simulink model "SR26_2024a"  (R2024a)
settings: Solver=FixedStepDiscrete  StartTime=0.0  StopTime=10.0  FixedStep=0.01  RelTol=1e-3  EnableMultiTasking=on
PreLoadFcn:
  | try, model_open; catch, disp('Error occurred while executing model pre-load callback: model_open.m'); disp('Please assure that the MATLAB working directory is set to the model directory before opening.'); end
InitFcn:
  | try, model_open; catch, end
values from neighbouring files (symbols this model uses):
  dt = 10.0    [SR26.sldd]
undefined symbols (not defined in the file or in its folder): GCM, raptor_get_safe_string, raptor_xcp_function
libraries: Raptor_lib x42, Utilities x6, simulink x5, IO x5, APPS_BSPC x4, Cooling x3, StateMachine x2, TorqueCommand x2, ATCC x2, BrakePressure x2, ThrottlePosition x2, Brakes x1
(part 1 of 2)
CloseFcn:
  | try, model_close; catch, end
settings Model: DataDictionary=SR26.sldd  Raptor_Target=GCM-1793-196-1503  Raptor_Calloc=NonVolatile (EEPROM)  RaptorUIDSize=4  RaptorBuildNum=0  Raptor_ecuaddr=11  RaptorFaultManager=Standard  RaptorFaultManagerAddXYCounts=1  Creator=hyuga  LastModifiedBy=hyuga
settings SolverCC: AlgebraicLoopSolver=TrustRegion
settings DataIOCC: LimitDataPoints=on  SaveFormat=Array  SignalLoggingSaveFormat=ModelDataLogs  ReturnWorkspaceOutputs=off
settings OptimizationCC: DefaultParameterBehavior=Inlined  ExpressionDepthLimit=2147483647  InitFltsAndDblsToZero=on  LifeSpan=1  EfficientTunableParamExpr=on
settings DebuggingCC: SolverPrmCheckMsg=warning  InheritedTsInSrcMsg=none  FcnCallInpInsideContextMsg=warning  UnconnectedInputMsg=warning  UnconnectedOutputMsg=warning  UnconnectedLineMsg=warning  StateNameClashWarn=warning  SFUnexpectedBacktrackingDiag=warning  SFNoUnconditionalDefaultTransitionDiag=warning  SFExecutionAtInitializationDiag=none  ArithmeticOperatorsInVariantConditions=warning
settings HardwareCC: ProdBitPerPointer=32  ProdBitPerSizeT=32  ProdBitPerPtrDiffT=32  ProdLargestAtomicFloat=None  ProdWordSize=32  ProdHWDeviceType=Infineon->TriCore  TargetBitPerPointer=64  TargetBitPerSizeT=64  TargetBitPerPtrDiffT=64  TargetLongLongMode=on  TargetIntDivRoundTo=Zero  TargetEndianess=LittleEndian  TargetWordSize=64  TargetHWDeviceType=MATLAB Host  ProdEqTarget=off
settings ModelReferenceCC: EnableRefExpFcnMdlSchedulingChecks=on  PropagateSignalLabelsOutOfModel=off
settings SFSimCC: SimUseLocalCustomCode=off  MATLABDynamicMemAlloc=off  CustomCodeUndefinedFunction=UseInterfaceOnly
settings RTWCC: Description=Raptor (tm)  SystemTargetFile=raptor.tlc  MakeCommand=raptor_make_rtw  TemplateMakefile=raptor.tmf  RTWUseLocalCustomCode=off  GPUComputeCapability=3.5  DLArmComputeVersion=19.05
settings CodeAppCC: IgnoreCustomStorageClasses=off  MaxIdLength=100  CustomSymbolStrType=$N$R$M  StateflowObjectComments=on  InternalIdentifier=Classic
settings STFCustomTargetCC: TargetLangStandard=C89/C90 (ANSI)  CodeReplacementLibrary=GCM196-specific  GenerateSampleERTMain=on  ModelReferenceCompliant=off  CombineOutputUpdateFcns=on  ERTCustomFileBanners=on  SupportContinuousTime=off  SupportNonInlinedSFcns=off  RemoveResetFunc=on  MATLABClassNameForMDSCustomization=Simulink.SoftwareTarget.ERTCustomization  GRTInterface=off  UseToolchainInfoCompliant=off  SystemTargetFile=raptor.tlc
settings ERTTargetCC: CodeReplacementLibrary=GCM196-specific  MultiwordLength=2048  GenerateSampleERTMain=on  ModelReferenceCompliant=off  ParMdlRefBuildCompliant=off  CompOptLevelCompliant=off  ConcurrentExecutionCompliant=off  ModelStepFunctionPrototypeControlCompliant=off  CPPClassGenCompliant=off  UseToolchainInfoCompliant=off  ExtModeMexFile=noextcomm  InlinedParameterPlacement=NonHierarchical  ERTCustomFileTemplate=example_file_process.tlc  ConvertIfToSwitch=off  SuppressUnreachableDefaultCases=off
settings ConfigComp: CovMetricSettings=dw  CovSaveCumulativeToWorkspaceVar=on  CovSaveSingleToWorkspaceVar=on  CovExternalEMLEnable=off  CovSFcnEnable=off  CovBoundaryAbsTol=1.0e-5

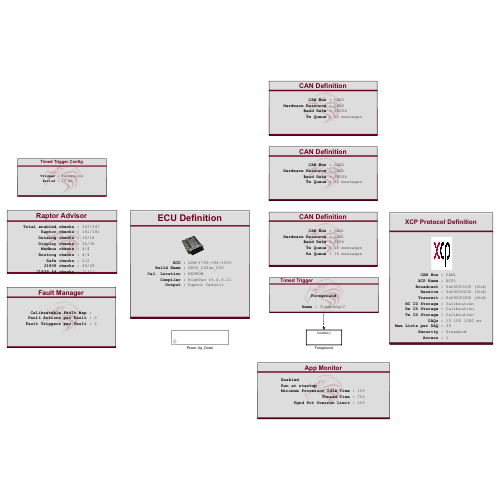
[thumbnail: Simulink's stored preview of the top-level diagram]
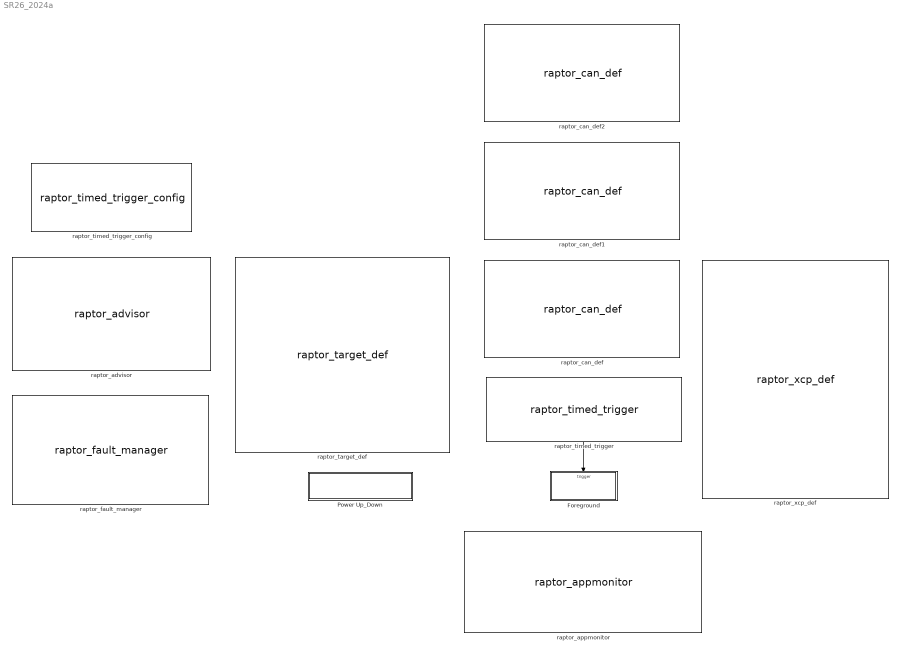
== system SR26_2024a ==
  Foreground : Subsystem  TreatAsAtomicUnit=on
      settings: RTWSystemCode=Nonreusable function
  Power Up_Down : Subsystem  mask{group='Diagnostics | Power Up_Down'}
  raptor_advisor : Raptor_lib/Configuration/raptor_advisor  pop_setEnable=Enable All  ckb_Raptor=on  ckb_AppMonitor=on  tbl_AppMonitor={ 'on', 'App Monitor'; 'on', 'App Monitor Measurement'; 'on', 'App Monitor Stop'; 'on', 'Reboot'; 'on', 'Task Monitor'; 'on', 'Task Monitor Measurement' }  ckb_CAN=on  tbl_CAN={ 'on', 'CAN Baud Rate'; 'on', 'CAN Bus Off Recovery'; 'on', 'CAN Definition'; 'on', 'CAN Hardware Mailbox Config'; 'on', 'CAN Mailbox Properties'; 'on', 'CAN Partial Networking'; 'on', 'CAN Queue Info'; 'on', 'CAN Rx Message'; 'on', 'CAN Rx Raw'; 'on', 'CAN State'; 'on', 'CAN Trigger'; 'on', 'CAN Tx Message'; 'on', 'CAN Tx Raw'; 'on', 'CAN/FD Definition'; 'on', 'CAN/FD Rx Message'; 'on', 'CAN/FD Rx Raw'; 'on', 'CAN/FD Tx Message'; 'on', 'CAN/FD Tx Raw'; 'on', 'Custom Baud Rate'; 'on', 'DBC Pack'; 'on', 'DBC Unpack' }  ckb_Checksum=on  tbl_Checksum={ 'on', 'Calculate Checksum'; 'on', 'Read Checksum' }  ckb_Config=on  tbl_Config={ 'on', 'Boot Request'; 'on', 'Configuration Read'; 'on', 'ECU Definition'; 'on', 'Set Target Address'; 'on', 'System Variable Access Level'; 'on', 'XCP Custom Security Seed/Key'; 'on', 'XCP Custom Security Trigger'; 'on', 'XCP Protocol Definition'; 'on', 'XCP Query'; 'on', 'XCP Set Address' }  ckb_DataStore=on  tbl_DataStore={ 'on', 'Adjustment'; 'on', 'Data Store'; 'on', 'Data Read'; 'on', 'Data Write'; 'on', 'Load NonVolatile Defaults'; 'on', 'Fixed NV Manager'; 'on', 'Measurement'; 'on', 'Memory Read'; 'on', 'NonVolatile Settings'; 'on', 'Override'; 'on', 'Fixed NonVolatile Status'; 'on', 'NonVolatile Status'; 'on', 'Store NonVolatile' }  ckb_Engine=on  tbl_Engine={ 'on', 'Angle Time'; 'on', 'CamShaft Sensor Info'; 'on', 'Encoder Def'; 'on', 'Injector Output'; 'on', 'Knock Results'; 'on', 'Knock Input'; 'on', 'Spark Output'; 'on', 'Wideband O2 Input' }  ckb_Ethernet=on  tbl_Ethernet={ 'on', 'Ethernet Adapter Get MAC Address'; 'on', 'Ethernet Definition'; 'on', 'Ethernet Hardware Info'; 'on', 'Ethernet Hardware Info Clear'; 'on', 'Ethernet Interface Definition'; 'on', 'Ethernet Interface Get VLAN'; 'on', 'Ethernet Interface Set VLAN'; 'on', 'Ethernet Socket - TCP Server'; 'on', 'Ethernet Socket - UDP Server'; 'on', 'Ethernet Socket State'; 'on', 'Ethernet TCP Accept'; 'on', 'Ethernet TCP Close'; 'on', 'Ethernet TCP Connect'; 'on', 'Ethernet TCP Listen'; 'on', 'Ethernet TCP Receive'; 'on', 'Ethernet TCP Send'; 'on', 'Ethernet TCP Shutdown'; 'on', 'Ethernet UDP Multicast Join'; 'on', 'Ethernet UDP Multicast Leave'; 'on', 'Ethernet UDP Receive'; 'on', 'Ethernet UDP Send'; 'on', 'PTP Get Epoch Time' }  ckb_OBD_Faults=on  tbl_OBD_Faults={ 'on', 'OBD Counter'; 'on', 'Increment OBD Counter'; 'on', 'Read OBD Counter'; 'on', 'Reset OBD Counter'; 'on', 'Drive Cycle Complete'; 'on', 'OBD Ratio'; 'on', 'Increment OBD Ratio'; 'on', 'Read OBD Ratio'; 'on', 'Reset OBD Ratio' }  ckb_Faults=on  tbl_Faults={ 'on', 'Fault Action'; 'on', 'Fault Action Iterator'; 'on', 'Fault Action Read'; 'on', 'Clear Fault'; 'on', 'Fault Data'; 'on', 'Fault Data Read'; 'on', 'Fault Data Write'; 'on', 'Fault'; 'on', 'Fault Handle'; 'on', 'Fault Iterator'; 'on', 'Fault Manager'; 'on', 'Fault Measurement'; 'on', 'Null Fault'; 'on', 'Fault Config'; 'on', 'Fault Reference'; 'on', 'Set Fault State'; 'on', 'Fault State Iterator'; 'on', 'Fault Status'; 'on', 'Fault Trigger'; 'on', 'Fault State Count' }  ckb_IO=on  tbl_IO={ 'on', 'Analog Input'; 'on', 'Analog Input Reference'; 'on', 'Analog Output'; 'on', 'Device Diagnostics'; 'on', 'Digital Input'; 'on', 'Digital Output'; 'on', 'Frequency Input'; 'on', 'H-Bridge Output'; 'on', 'IMU Calibrate'; 'on', 'IMU Reset'; 'on', 'IMU Status'; 'on', 'Inertial Measurement'; 'on', 'Input Capture Defn'; 'on', 'Input Capture Get'; 'on', 'Input Capture Trigger'; 'on', 'Input Status'; 'on', 'Internal Measurement'; 'on', 'Output Status'; 'on', 'PWM Output'; 'on', 'Quadrature Input'; 'on', 'Set Hardware Option'; 'on', 'Set Input Option'; 'on', 'Temperature Measurement' }  ckb_LIN=on  tbl_LIN={ 'on', 'LIN Master Definition'; 'on', 'LIN Get Schedule'; 'on', 'LIN Rx Message'; 'on', 'LIN Set Schedule'; 'on', 'LIN Slave Definition'; 'on', 'LIN State'; 'on', 'LIN Trigger'; 'on', 'LIN Tx Message' }  ckb_SENT=on  tbl_SENT={ 'on', 'SENT Definition'; 'on', 'SENT Receive State' }  ckb_Serial=on  tbl_Serial={ 'on', 'Serial Definition'; 'on', 'Serial Rx'; 'on', 'Serial Trigger'; 'on', 'Serial Tx' }  ckb_Strings=on  tbl_Strings={ 'on', 'String'; 'on', 'Arr 2 Str'; 'on', 'String Length'; 'on', 'Printf'; 'on', 'String Reference'; 'on', 'scanf'; 'on', 'Str 2 Arr' }  ckb_Tables=on  tbl_Tables={ 'on', 'Table Adapt'; 'on', 'Axis'; 'on', 'Axis Reference'; 'on', 'Table Interpolate 1D'; 'on', 'Table Interpolate 1D Reference'; 'on', 'Table Interpolate 2D'; 'on', 'Table Interpolate 2D Reference' }  ckb_Time=on  tbl_Time={ 'on', 'Datetime Conversion In'; 'on', 'Datetime Conversion Out'; 'on', 'Real Time Clock Read'; 'on', 'Real Time Clock Set' }  ckb_Triggers=on  tbl_Triggers={ 'on', 'App Trigger'; 'on', 'dT'; 'on', 'Distributed Action Defn'; 'on', 'Distributed Action Execute'; 'on', 'Distributed Action Trigger'; 'on', 'Shutdown'; 'on', 'Sleep'; 'on', 'Startup'; 'on', 'Time'; 'on', 'Timed Trigger'; 'on', 'Timed Trigger Config'; 'on', 'Define Trigger'; 'on', 'Trigger Execute'; 'on', 'Output Trigger Reference'; 'on', 'Trigger Select' }  ckb_DataLog=on  tbl_DataLog={ 'on', 'Data Log Erase'; 'on', 'Data Log Read'; 'on', 'Data Log Write'; 'on', 'File Close'; 'on', 'File EOF'; 'on', 'File Exists'; 'on', 'File Get Free Space'; 'on', 'File Open'; 'on', 'File Position'; 'on', 'File Read'; 'on', 'File Remove'; 'on', 'File Rename'; 'on', 'File Seek'; 'on', 'File Size'; 'on', 'File Sync'; 'on', 'USB Eject'; 'on', 'USB Status'; 'on', 'File Write' }  ckb_Display=on  ckb_Drawing=on  tbl_Drawing={ 'on', 'Clear Rect'; 'on', 'Clear Screen'; 'on', 'Draw Arc'; 'on', 'Draw Button'; 'on', 'Draw Circle'; 'on', 'Draw Image'; 'on', 'Draw Line'; 'on', 'Draw Polygon'; 'on', 'Draw Rectangle'; 'on', 'Draw Text'; 'on', 'Element'; 'on', 'Fill Circle'; 'on', 'Fill Ellipse'; 'on', 'Fill Polygon'; 'on', 'Fill Rect'; 'on', 'Image Ref' }  ckb_Menu=on  tbl_Menu={ 'on', 'Menu Screen Definition'; 'on', 'Menu Sel Item'; 'on', 'Menu Text'; 'on', 'Menu Title' }  ckb_Prefab=on  tbl_Prefab={ 'on', 'Gauge: Create'; 'on', 'Gauge: Update' }  ckb_ScreenFuncs=on  tbl_ScreenFuncs={ 'on', 'Hide Buttonbar'; 'on', 'Button Bar Properties'; 'on', 'Setup Button'; 'on', 'Goto Screen'; 'on', 'Recalibrate Screen'; 'on', 'Screen Definition'; 'on', 'Screen Reference'; 'on', 'Screen Select'; 'on', 'Splash Screen' }  ckb_Touchscreen=on  tbl_Touchscreen={ 'on', 'Button Status'; 'on', 'Display Touchscreen'; 'on', 'Button Def'; 'on', 'Hot Area Actions'; 'on', 'Update Swipe Action' }  ckb_Modbus=on  tbl_Modbus={ 'on', 'Modbus Master'; 'on', 'Modbus Slave'; 'on', 'Modbus Slave Error'; 'on', 'Modbus Slave Response' }  ckb_Routing=on  tbl_Routing={ 'on', 'J1939 Message Router'; 'on', 'Message Hardware Filter'; 'on', 'Message Network'; 'on', 'Message Router' }  ckb_Safe=on  tbl_Safe={ 'on', 'Raptor Stack Check'; 'on', 'Raptor Time Check' }  ckb_J1939=on  ckb_DMA=on  tbl_DMA={ 'on', 'DM14/15/16 Definition: DM14 Rx'; 'on', 'DM14/15/16 Definition: DM15 Rx'; 'on', 'DM14/15/16 Definition: DM15 Tx'; 'on', 'DM14/15/16 Definition: DMA Manager'; 'on', 'DMA Address Space Definition'; 'on', 'DMA Address Space Return'; 'on', 'DMA Address Space Trigger'; 'on', 'DMA Key'; 'on', 'DMA Key Trigger' }  ckb_DM_Msgs=on  tbl_DM_Msgs={ 'on', 'DM4 Transmit'; 'on', 'DM5 Transmit'; 'on', 'DM8 Transmit'; 'on', 'DM19 Transmit'; 'on', 'DM20 Transmit'; 'on', 'DM21 Transmit'; 'on', 'DM22 Rx Trigger'; 'on', 'DM24 Transmit'; 'on', 'DM25 Transmit'; 'on', 'DM26 Transmit'; 'on', 'DM29 Transmit'; 'on', 'DM30 Transmit'; 'on', 'DM33 Transmit'; 'on', 'DM34 Transmit'; 'on', 'DTC Transmit' }  ckb_EFF=on  tbl_EFF={ 'on', 'Clear Expanded FF'; 'on', 'Write Expanded FF'; 'on', 'Expanded FF Status' }  ckb_PGN_Tx=on  tbl_PGN_Tx={ 'on', 'CBI Transmit'; 'on', 'CI Transmit'; 'on', 'EC1 Transmit'; 'on', 'ECUID Transmit'; 'on', 'GTFI Transmit'; 'on', 'LTFI Transmit'; 'on', 'RC Transmit'; 'on', 'SOFT Transmit'; 'on', 'TTI2 Transmit'; 'on', 'VI Transmit' }  ckb_SPN=on  tbl_SPN={ 'on', 'SPN Read'; 'on', 'SPN Write' }  ckb_J1939_TP=on  tbl_J1939_TP={ 'on', 'J1939 DTC Rx Handler'; 'on', 'Source Addr'; 'on', 'PGN Enable'; 'on', 'PGN Request Slot'; 'on', 'PGN Enable'; 'on', 'PGN Trigger'; 'on', 'Tx ACK/NACK'; 'on', 'J1939 Protocol'; 'on', 'J1939 Transport Protocol Receive'; 'on', 'PGN Rx Trigger' }  ckb_J1939_fd=on  ckb_J1939_fd_TP=on  tbl_J1939_fd_TP={'on','Get J1939 STD/FD Channel Addr.';'on','Rx Raw';'on','Transport Protocol';'on','Tx Raw'}  ckb_J1939_fd_GW=on  tbl_J1939_fd_GW={ 'on', 'Gateway'; 'on', 'Gateway Link'; 'on', 'Gateway Link Reset Stats'; 'on', 'Gateway Link Stats'; 'on', 'Gateway Network' }  ckb_UDS=on  ckb_ISO14229=on  tbl_ISO14229={ 'on', 'ISO14229 Custom Service 0x31'; 'on', 'ISO14229 Service 0x10 - Session Control'; 'on', 'ISO14229 Service 0x11 - ECU Reset'; 'on', 'ISO14229 Service 0x14 - Clear Diagnostic Information'; 'on', 'ISO14229 Service 0x19 - Read DTC Information'; 'on', 'ISO14229 Service 0x19 - Extended Data Definition'; 'on', 'ISO14229 Service 0x19 - Snapshot Record Definition'; 'on', 'ISO14229 Service 0x19 - Snapshot Record Clear'; 'on', 'ISO14229 Service 0x19 - Snapshot Record Clear All'; 'on', 'ISO14229 Service 0x19 - Snapshot Record Get'; 'on', 'ISO14229 Service 0x19 - Snapshot Record Set'; 'on', 'ISO14229 Service 0x22 - Read Data by Identifier'; 'on', 'ISO14229 Service 0x27 - Security Access'; 'on', 'ISO14229 Service 0x28 - Communication Control'; 'on', 'ISO14229 Service 0x2E - Write Data by Identifier'; 'on', 'ISO14229 Service 0x2F - Input Output by Identifier'; 'on', 'ISO14229 Service 0x2F - Input Output by Identifier Reset State'; 'on', 'ISO14229 Service 0x31 - Routine Control by Identifier'; 'on', 'ISO14229 Service 0x85 - DTC Control Setting' }  ckb_ISO15031=on  tbl_ISO15031={ 'on', 'ISO15031 Custom Service'; 'on', 'ISO15031 Service 0x01'; 'on', 'ISO15031 Service 0x03 - Emission-related diagnostic trouble codes'; 'on', 'ISO15031 Service 0x04 - Clear Diagnostic Information'; 'on', 'ISO15031 Service 0x07 - Emission-related pending diagnostic trouble codes'; 'on', 'ISO15031 Service 0x09 - Calibration Identification'; 'on', 'ISO15031 Service 0x09 - Calibration Verification Numbers'; 'on', 'ISO15031 Service 0x09 - ECU Name'; 'on', 'ISO15031 Service 0x09 - Request Vehicle Information'; 'on', 'ISO15031 Service 0x09 - Vehicle Identification Number'; 'on', 'ISO15031 Service 0x0A - Emission-related diagnostic trouble codes with permanent status' }  ckb_ISO15765=on  tbl_ISO15765={ 'on', 'ISO15765 Protocol Receive Queue Info'; 'on', 'ISO15765 Protocol Transmit Queue Info'; 'on', 'ISO15765 Protocol Transmit Raw' }  ckb_UDS_Basics=on  tbl_UDS_Basics={ 'on', 'UDS Client Functional Address Request'; 'on', 'UDS Client Functional Address Request Send'; 'on', 'UDS Protocol Client Request Raw'; 'on', 'UDS Protocol Receive Raw'; 'on', 'UDS Protocol Transmit Raw'; 'on', 'UDS Server Service Process Raw' }  ckb_UDS_Other=on  tbl_UDS_Other={ 'on', 'ISO13400 DoIP Entity'; 'on', 'UDS Protocol'; 'on', 'UDS Set Buffer Storage' }  ckb_J1939_Assure=on  tbl_J1939_Assure={ 'on', 'J1939-91C Network Config'; 'on', 'J1939-91C Network State' }
      settings: SourceProductName=Raptor
  raptor_appmonitor : Raptor_lib/Application Monitoring/raptor_appmonitor  enabled=on  startupAction=Run  addStartupActionCal=off  minIdle=10  maxThread=70  calAccess=1  pctOverrunLimit=20  overrunAction=Stop Application  pauseOnReset=on  maxStackUsage=90  stackOverrunAction=Stop Application  addMaxStackCal=off  CANen=off
      settings: SourceProductName=Raptor
  raptor_can_def : Raptor_lib/CAN/raptor_can_def  canBus='CAN1'  resourceValues=(None)|CAN1|CAN2  resource=CAN1  baudRateValues=250k  baudRate=250k  useCustomBR=0  customBR='CustomBaudRate'  enable_baud_rate_config='RAPTOR MASK DEFAULT'  sim_func_name='RAPTOR MASK DEFAULT'  createButton=[]  updateButton=[]  txQueueSize=16  rxQueueSize=16
      settings: SourceProductName=Raptor
  raptor_can_def1 : Raptor_lib/CAN/raptor_can_def  canBus='CAN2'  resourceValues=CAN1|CAN2|CAN3|(None)  resource=CAN2  baudRateValues=125k|250k|500k|1000k  baudRate=1000k  useCustomBR=0  customBR='CustomBaudRate'  enable_baud_rate_config='RAPTOR MASK DEFAULT'  sim_func_name='RAPTOR MASK DEFAULT'  createButton=[]  updateButton=[]  txQueueSize=25  rxQueueSize=16
      settings: SourceProductName=Raptor
  raptor_can_def2 : Raptor_lib/CAN/raptor_can_def  canBus='CAN3'  resourceValues=CAN1|CAN2|CAN3|(None)  resource=CAN3  baudRateValues=125k|250k|500k|1000k  baudRate=1000k  useCustomBR=0  customBR='CustomBaudRate'  enable_baud_rate_config='RAPTOR MASK DEFAULT'  sim_func_name='RAPTOR MASK DEFAULT'  createButton=[]  updateButton=[]  txQueueSize=25  rxQueueSize=16
      settings: SourceProductName=Raptor
  raptor_fault_manager : Raptor_lib/Faults/raptor_fault_manager  button=[]  managerTypeValues=Standard|OBD  managerType=Standard  cyclesToHeal=3  cyclesToClear=40  addXYCounts=1  calFaultMap=1  minFaultActions=2  minFaultTriggers=2  calAccessValues=4|3|2|1  calAccess=1  calFunction='System | FaultManager'  initMap=struct()  exportFilePath='C:\'  exportFileName='FaultMapExport_01.csv'
      settings: SourceProductName=Raptor
  raptor_target_def : Raptor_lib/Configuration/raptor_target_def  targetValues=HCM-5534-50-1203|HCM-5534-90-1201|HCM-5534-90-1302|HCM-5604-36-1303|HCM-ARM4-070-1401|DISP-IMX286-036-1402|DISP-IMX286-024-1204|DISP-IMX286-012-1402  target=GCM-1793-196-1503  simpack=0  simulator=0  heap=4*1024  stack=2*1024  fgndStack=3*1024  bgndStack=2*1024  idleStack=1024  intStack=1536  sdStack=1024  appStack=1024  ecuaddr=11  disable_def_uds_reflash=0  uds_server_addr_ext=0  uds_server_addr=hex2dec('600')  uds_client_addr=hex2dec('650')  callocValues=Constant (FLASH)|NonVolatile (EEPROM)  calloc=NonVolatile (EEPROM)  compilerValues=[]  compiler=HighTec v3.4.5.11  setFileName=0  exeName=[raptor_get_safe_string(bdroot) '_']  addBuildNum=1  minVerChars=3  extraOutput=0  buildLocationValues=Raptor Default|Model Directory|User Defined  buildLocation=Raptor Default  exeLocation=''  exeFileButton=[]  a2lLocation=''  a2lFileButton=[]  rpgLocation=''  rpgFileButton=[]
      settings: SourceProductName=Raptor
  raptor_timed_trigger : Raptor_lib/Triggers/raptor_timed_trigger  triggerValues=[]  trigger=Foreground  inherited=0  alwaysEnabled=1  triggerPriority=0  triggerName=ooqlV
      settings: SourceProductName=Raptor
  raptor_timed_trigger_config : Raptor_lib/Triggers/raptor_timed_trigger_config  triggerValues=Foreground|Background|Second|Minute  trigger=Foreground  period=10
      settings: SourceProductName=Raptor
  raptor_xcp_def : Raptor_lib/Configuration/raptor_xcp_def  XCPname='XCP1'  canBus='CAN1'  bcID=hex2dec('100')  bcID_TypeValues=Standard|Extended  bcID_Type=Standard  rxID=hex2dec('200')  rxID_TypeValues=Standard|Extended  rxID_Type=Standard  txID=hex2dec('300')  txID_TypeValues=Standard|Extended  txID_Type=Standard  daqRates=[10 100 1000]  numODTs=30  genCANAPE=0  genVISION=0  securityValues=Standard|None|Custom User Defined  security=Standard  dllName=raptor_XCPSecurity.dll  accessValues=4|3|2|1  access=1  bcStorageValues=Constant (FLASH)|NonVolatile (EEPROM)|FixedNonVolatile (EEPROM)|Volatile (RAM)|Calibration  bcStorage=Calibration  txStorageValues=Constant (FLASH)|NonVolatile (EEPROM)|FixedNonVolatile (EEPROM)|Volatile (RAM)|Calibration  txStorage=Calibration  rxStorageValues=Constant (FLASH)|NonVolatile (EEPROM)|FixedNonVolatile (EEPROM)|Volatile (RAM)|Calibration  rxStorage=Calibration
      settings: SourceProductName=Raptor
  wires:
  raptor_timed_trigger/1 -> Foreground/Trigger

== system SR26_2024a/Foreground ==
  function : TriggerPort  TriggerType=function-call  VariantControl=Variant
  Add : Sum  Commented=on
  Constant : Constant  Commented=on
  Controls Algorithm : Subsystem
  IO : Subsystem
  InputProcessing : Subsystem
  OutputProcessing : Subsystem
  Unit Delay : UnitDelay  Commented=on  SampleTime=-1  HasFrameUpgradeWarning=on
  raptor_measurement : Raptor_lib/Data Storage/raptor_measurement  Commented=on  paramName='Counter'  nameSource=Parameter  calDispType=Number  calEnum={'False', 'True'}  calGain=1.0  calOffset=0.0  calMax=inf  calMin=-inf  calFormat='-1'  calUnit=''  calHelp=''  calAccess=4  calFunction=raptor_xcp_function(gcb)  calVisible=on
      settings: SourceProductName=Raptor
  wires:
  Constant/1 -> Add/1
  Add/1 -> raptor_measurement/1, Unit Delay/1
  Unit Delay/1 -> Add/2
  IO/1(IO_Inputs_Bus) -> OutputProcessing/1(IO_Inputs_Bus), Controls Algorithm/1(IO_Inputs_Bus), InputProcessing/1(IO_Inputs_Bus)
  InputProcessing/1(IN_Inputs_Bus) -> OutputProcessing/3(IN_Inputs_Bus), Controls Algorithm/2(IN_Inputs_Bus)
  Controls Algorithm/1(CTRL_Controls_Bus) -> OutputProcessing/2(CTRL_Controls_Bus)
  OutputProcessing/1(IO_Outputs_Bus) -> IO/1(IO_Outputs_Bus)

== system SR26_2024a/Power Up_Down ==
  Background : Subsystem
  raptor_timed_trigger : Raptor_lib/Triggers/raptor_timed_trigger  triggerValues=Foreground|Foregroundx2|Foregroundx5|Foregroundx10|Foregroundx20|Background|Backgroundx2|Backgroundx5|Backgroundx10|Backgroundx20|Second|Minute  trigger=Background  inherited=0  alwaysEnabled=1  triggerPriority=50  triggerName=BGND_G6Wyo
      settings: SourceProductName=Raptor
  wires:
  raptor_timed_trigger/1 -> Background/Trigger

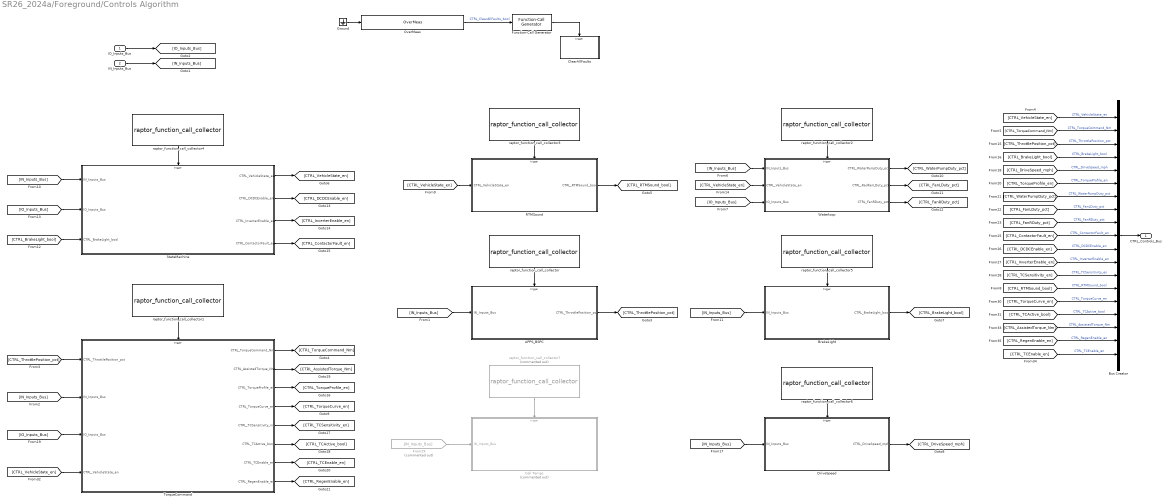
== system SR26_2024a/Foreground/Controls Algorithm ==
  IO_Inputs_Bus : Inport
  IN_Inputs_Bus : Inport  Port=2
  APPS_BSPC : Subsystem
  BrakeLight : Subsystem
  Bus Creator : BusCreator  Inputs=19
  Cell Temps : Subsystem  Commented=on
  ClearAllFaults : Subsystem  TreatAsAtomicUnit=on
  DriveSpeed : Subsystem
  From29 : From  Commented=on  GotoTag=IN_Inputs_Bus
  Function-Call Generator : simulink/Ports & Subsystems/Function-Call Generator  sample_time=1  numberOfIterations=1  DisallowWideOutput=off  ShowEnablePort=on
  Ground : Ground
  OverMeas : Utilities/OverMeas  sigName='CTRL_ClearAllFaults_bool'  minimum=-inf  maximum=inf
  RTMSound : Subsystem
  StateMachine : Subsystem
  TorqueCommand : Subsystem
  Waterloop : Subsystem
  raptor_function_call_collector{,1,3..4} (4 alike) : Raptor_lib/Triggers/raptor_function_call_collector  count=1
      settings: SourceProductName=Raptor
  raptor_function_call_collector2 : Raptor_lib/Triggers/raptor_function_call_collector  count=100
      settings: SourceProductName=Raptor
  raptor_function_call_collector5 : Raptor_lib/Triggers/raptor_function_call_collector  count=10
      settings: SourceProductName=Raptor
  raptor_function_call_collector6 : Raptor_lib/Triggers/raptor_function_call_collector  count=10
      settings: SourceProductName=Raptor
  raptor_function_call_collector7 : Raptor_lib/Triggers/raptor_function_call_collector  Commented=on  count=100
      settings: SourceProductName=Raptor
  CTRL_Controls_Bus : Outport
  wires:
  IO_Inputs_Bus/1 -> [IO_Inputs_Bus]
  IN_Inputs_Bus/1 -> [IN_Inputs_Bus]
  OverMeas/1 -> Function-Call Generator/1  "CTRL_ClearAllFaults_bool"
  Ground/1 -> OverMeas/1
  Function-Call Generator/1 -> ClearAllFaults/Trigger
  [IN_Inputs_Bus] -> APPS_BSPC/1(IN_Inputs_Bus)
  APPS_BSPC/1(CTRL_ThrottlePosition_pct) -> [CTRL_ThrottlePosition_pct]
  raptor_function_call_collector/1 -> APPS_BSPC/Trigger
  raptor_function_call_collector1/1 -> TorqueCommand/Trigger
  TorqueCommand/1(CTRL_TorqueCommand_Nm) -> [CTRL_TorqueCommand_Nm]
  [IN_Inputs_Bus] -> TorqueCommand/2(IN_Inputs_Bus)
  [CTRL_ThrottlePosition_pct] -> TorqueCommand/1(CTRL_ThrottlePosition_pct)
  Bus Creator/1 -> CTRL_Controls_Bus/1
  [CTRL_VehicleState_en] -> Bus Creator/1  "CTRL_VehicleState_en"
  [CTRL_TorqueCommand_Nm] -> Bus Creator/2  "CTRL_TorqueCommand_Nm"
  raptor_function_call_collector2/1 -> Waterloop/Trigger
  [IN_Inputs_Bus] -> Waterloop/1(IN_Inputs_Bus)
  [IO_Inputs_Bus] -> Waterloop/3(IO_Inputs_Bus)
  RTMSound/1(CTRL_RTMSound_bool) -> [CTRL_RTMSound_bool]
  [CTRL_VehicleState_en] -> RTMSound/1(CTRL_VehicleState_en)
  raptor_function_call_collector3/1 -> RTMSound/Trigger
  raptor_function_call_collector4/1 -> StateMachine/Trigger
  StateMachine/1(CTRL_VehicleState_en) -> [CTRL_VehicleState_en]
  [IN_Inputs_Bus] -> StateMachine/1(IN_Inputs_Bus)
  BrakeLight/1(CTRL_BrakeLight_bool) -> [CTRL_BrakeLight_bool]
  [IN_Inputs_Bus] -> BrakeLight/1(IN_Inputs_Bus)
  raptor_function_call_collector5/1 -> BrakeLight/Trigger
  [CTRL_BrakeLight_bool] -> StateMachine/3(CTRL_BrakeLight_bool)
  [IO_Inputs_Bus] -> StateMachine/2(IO_Inputs_Bus)
  [CTRL_VehicleState_en] -> Waterloop/2(CTRL_VehicleState_en)
  [CTRL_ThrottlePosition_pct] -> Bus Creator/3  "CTRL_ThrottlePosition_pct"
  [CTRL_BrakeLight_bool] -> Bus Creator/4  "CTRL_BrakeLight_bool"
  raptor_function_call_collector6/1 -> DriveSpeed/Trigger
  [IN_Inputs_Bus] -> DriveSpeed/1(IN_Inputs_Bus)
  DriveSpeed/1(CTRL_DriveSpeed_mph) -> [CTRL_DriveSpeed_mph]
  [CTRL_DriveSpeed_mph] -> Bus Creator/5  "CTRL_DriveSpeed_mph"
  [IO_Inputs_Bus] -> TorqueCommand/3(IO_Inputs_Bus)
  TorqueCommand/4(CTRL_TorqueCurve_en) -> [CTRL_TorqueCurve_en]
  [CTRL_TorqueProfile_en] -> Bus Creator/6  "CTRL_TorqueProfile_en"
  Waterloop/1(CTRL_WaterPumpDuty_pct) -> [CTRL_WaterPumpDuty_pct]
  Waterloop/2(CTRL_RadFanLDuty_pct) -> [CTRL_FanLDuty_pct]
  Waterloop/3(CTRL_FanRDuty_pct) -> [CTRL_FanRDuty_pct]
  [CTRL_WaterPumpDuty_pct] -> Bus Creator/7  "CTRL_WaterPumpDuty_pct"
  [CTRL_FanLDuty_pct] -> Bus Creator/8  "CTRL_FanLDuty_pct"
  [CTRL_FanRDuty_pct] -> Bus Creator/9  "CTRL_FanRDuty_pct"
  StateMachine/2(CTRL_DCDCEnable_en) -> [CTRL_DCDCEnable_en]
  StateMachine/3(CTRL_InverterEnable_en) -> [CTRL_InverterEnable_en]
  StateMachine/4(CTRL_ContactorFault_en) -> [CTRL_ContactorFault_en]
  From29/1 -> Cell Temps/1(IN_Inputs_Bus)
  raptor_function_call_collector7/1 -> Cell Temps/Trigger
  TorqueCommand/3(CTRL_TorqueProfile_en) -> [CTRL_TorqueProfile_en]
  TorqueCommand/5(CTRL_TCSensitivity_int) -> [CTRL_TCSensitivity_en]
  [CTRL_VehicleState_en] -> TorqueCommand/4(CTRL_VehicleState_en)
  TorqueCommand/2(CTRL_AssistedTorque_Nm) -> [CTRL_AssistedTorque_Nm]
  TorqueCommand/6(CTRL_TCActive_bool) -> [CTRL_TCActive_bool]
  [CTRL_ContactorFault_en] -> Bus Creator/10  "CTRL_ContactorFault_en"
  [CTRL_DCDCEnable_en] -> Bus Creator/11  "CTRL_DCDCEnable_en"
  [CTRL_InverterEnable_en] -> Bus Creator/12  "CTRL_InverterEnable_en"
  [CTRL_TCSensitivity_en] -> Bus Creator/13  "CTRL_TCSensitivity_en"
  [CTRL_RTMSound_bool] -> Bus Creator/14  "CTRL_RTMSound_bool"
  [CTRL_TorqueCurve_en] -> Bus Creator/15  "CTRL_TorqueCurve_en"
  [CTRL_TCActive_bool] -> Bus Creator/16  "CTRL_TCActive_bool"
  [CTRL_AssistedTorque_Nm] -> Bus Creator/17  "CTRL_AssistedTorque_Nm"
  TorqueCommand/7(CTRL_TCEnable_en) -> [CTRL_TCEnable_en]
  TorqueCommand/8(CTRL_RegenEnable_en) -> [CTRL_RegenEnable_en]
  [CTRL_TCEnable_en] -> Bus Creator/19  "CTRL_TCEnable_en"
  [CTRL_RegenEnable_en] -> Bus Creator/18  "CTRL_RegenEnable_en"

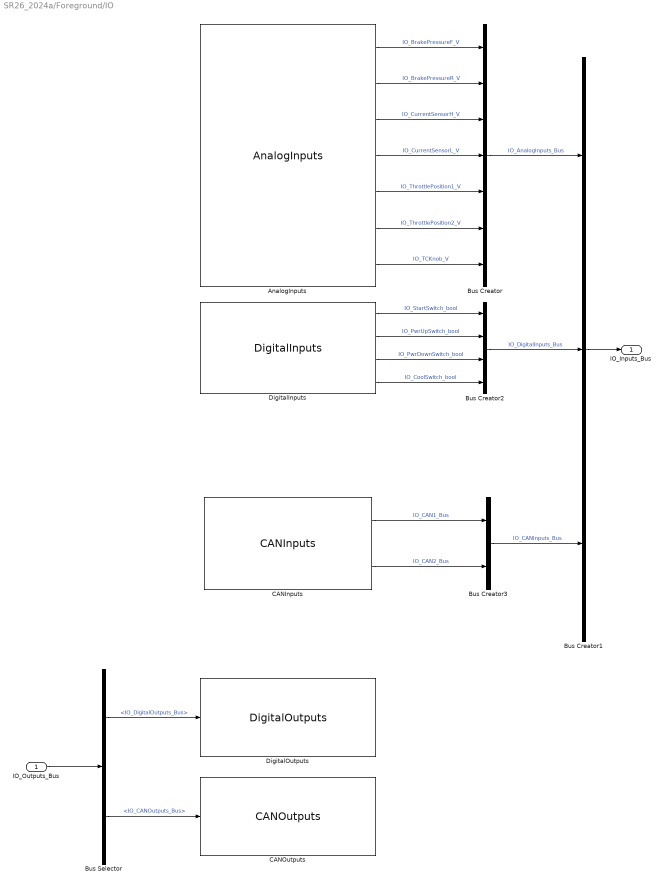
== system SR26_2024a/Foreground/IO ==
  IO_Outputs_Bus : Inport
  AnalogInputs : IO/AnalogInputs  SystemSampleTime=-1  VariantActivationTime=update diagram  EmptyChoice=off  PassThrough=off  PassThroughVariantControl=(default)  EmptyChoiceVariantControl=(default)  AllowFlexibleInterface=on  Latency=0  AutoFrameSizeCalculation=off
  Bus Creator : BusCreator  Inputs=7
  Bus Creator1 : BusCreator  Inputs=3
  Bus Creator2 : BusCreator  Inputs=4
  Bus Creator3 : BusCreator  Inputs=2
  Bus Selector : BusSelector  OutputSignals=IO_DigitalOutputs_Bus,IO_CANOutputs_Bus
  CANInputs : IO/CANInputs  SystemSampleTime=-1  VariantActivationTime=update diagram  EmptyChoice=off  PassThrough=off  PassThroughVariantControl=(default)  EmptyChoiceVariantControl=(default)  AllowFlexibleInterface=on  Latency=0  AutoFrameSizeCalculation=off
  CANOutputs : IO/CANOutputs  SystemSampleTime=-1  VariantActivationTime=update diagram  EmptyChoice=off  PassThrough=off  PassThroughVariantControl=(default)  EmptyChoiceVariantControl=(default)  AllowFlexibleInterface=on  Latency=0  AutoFrameSizeCalculation=off
  DigitalInputs : IO/DigitalInputs  SystemSampleTime=-1  VariantActivationTime=update diagram  EmptyChoice=off  PassThrough=off  PassThroughVariantControl=(default)  EmptyChoiceVariantControl=(default)  AllowFlexibleInterface=on  Latency=0  AutoFrameSizeCalculation=off
  DigitalOutputs : IO/DigitalOutputs  SystemSampleTime=-1  VariantActivationTime=update diagram  EmptyChoice=off  PassThrough=off  PassThroughVariantControl=(default)  EmptyChoiceVariantControl=(default)  AllowFlexibleInterface=on  Latency=0  AutoFrameSizeCalculation=off
  IO_Inputs_Bus : Outport
  wires:
  DigitalInputs/2 -> Bus Creator2/2  "IO_PwrUpSwitch_bool"
  Bus Creator1/1 -> IO_Inputs_Bus/1
  DigitalInputs/3 -> Bus Creator2/3  "IO_PwrDownSwitch_bool"
  DigitalInputs/4 -> Bus Creator2/4  "IO_CoolSwitch_bool"
  AnalogInputs/1 -> Bus Creator/1  "IO_BrakePressureF_V"
  AnalogInputs/2 -> Bus Creator/2  "IO_BrakePressureR_V"
  AnalogInputs/3 -> Bus Creator/3  "IO_CurrentSensorH_V"
  AnalogInputs/4 -> Bus Creator/4  "IO_CurrentSensorL_V"
  AnalogInputs/7 -> Bus Creator/7  "IO_TCKnob_V"
  AnalogInputs/6 -> Bus Creator/6  "IO_ThrottlePosition2_V"
  AnalogInputs/5 -> Bus Creator/5  "IO_ThrottlePosition1_V"
  Bus Creator/1 -> Bus Creator1/1  "IO_AnalogInputs_Bus"
  Bus Creator2/1 -> Bus Creator1/2  "IO_DigitalInputs_Bus"
  DigitalInputs/1 -> Bus Creator2/1  "IO_StartSwitch_bool"
  CANInputs/1 -> Bus Creator3/1  "IO_CAN1_Bus"
  CANInputs/2 -> Bus Creator3/2  "IO_CAN2_Bus"
  Bus Creator3/1 -> Bus Creator1/3  "IO_CANInputs_Bus"
  IO_Outputs_Bus/1 -> Bus Selector/1
  Bus Selector/1 -> DigitalOutputs/1  "<IO_DigitalOutputs_Bus>"
  Bus Selector/2 -> CANOutputs/1  "<IO_CANOutputs_Bus>"

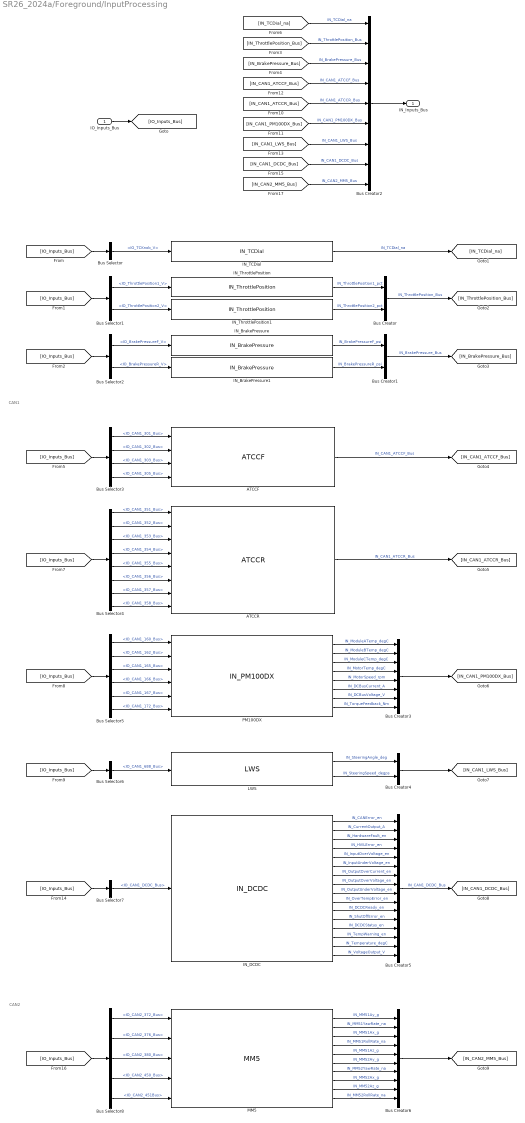
== system SR26_2024a/Foreground/InputProcessing ==
  note: CAN2
  note: CAN1
  IO_Inputs_Bus : Inport
  ATCCF : ATCC/ATCCF  SystemSampleTime=-1  VariantActivationTime=update diagram  EmptyChoice=off  PassThrough=off  PassThroughVariantControl=(default)  EmptyChoiceVariantControl=(default)  AllowFlexibleInterface=on  Latency=0  AutoFrameSizeCalculation=off
  ATCCR : ATCC/ATCCR  SystemSampleTime=-1  VariantActivationTime=update diagram  EmptyChoice=off  PassThrough=off  PassThroughVariantControl=(default)  EmptyChoiceVariantControl=(default)  AllowFlexibleInterface=on  Latency=0  AutoFrameSizeCalculation=off
  Bus Creator : BusCreator  Inputs=2
  Bus Creator1 : BusCreator  Inputs=2
  Bus Creator2 : BusCreator  Inputs=9
  Bus Creator3 : BusCreator  Inputs=8
  Bus Creator4 : BusCreator  Inputs=2
  Bus Creator5 : BusCreator  Inputs=16
  Bus Creator6 : BusCreator  Inputs=10
  Bus Selector : BusSelector  OutputSignals=IO_AnalogInputs_Bus.IO_TCKnob_V
  Bus Selector1 : BusSelector  OutputSignals=IO_AnalogInputs_Bus.IO_ThrottlePosition1_V,IO_AnalogInputs_Bus.IO_ThrottlePosition2_V
  Bus Selector2 : BusSelector  OutputSignals=IO_AnalogInputs_Bus.IO_BrakePressureF_V,IO_AnalogInputs_Bus.IO_BrakePressureR_V
  Bus Selector3 : BusSelector  OutputSignals=IO_CANInputs_Bus.IO_CAN1_Bus.IO_CAN1_ATCCF_Bus.IO_CAN1_301_Bus,IO_CANInputs_Bus.IO_CAN1_Bus.IO_CAN1_ATCCF_Bus.IO_CAN1_302_Bus,IO_CANInputs_Bus.IO_CAN1_Bus.IO_CAN1_ATCCF_Bus.IO_CAN1_303_Bus,IO_CANInputs_Bus.IO_CAN1_Bus.IO_CAN1_ATCCF_Bus.IO_CAN1_305_Bus
  Bus Selector4 : BusSelector  OutputSignals=IO_CANInputs_Bus.IO_CAN1_Bus.IO_CAN1_ATCCR_Bus.IO_CAN1_351_Bus,IO_CANInputs_Bus.IO_CAN1_Bus.IO_CAN1_ATCCR_Bus.IO_CAN1_352_Bus,IO_CANInputs_Bus.IO_CAN1_Bus.IO_CAN1_ATCCR_Bus.IO_CAN1_353_Bus,IO_CANInputs_Bus.IO_CAN1_Bus.IO_CAN1_ATCCR_Bus.IO_CAN1_354_Bus,IO_CANInputs_Bus.IO_CAN1_Bus.IO_CAN1_ATCCR_Bus.IO_CAN1_355_Bus,IO_CANInputs_Bus.IO_CAN1_Bus.IO_CAN1_ATCCR_Bus.IO_CAN1_356_Bus,IO_CANInputs_Bus.IO_CAN1_Bus.IO_CAN1_ATCCR_Bus.IO_CAN1_357_Bus,IO_CANInputs_Bus.IO_CAN1_Bus.IO_CAN1_ATCCR_Bus.IO_CAN1_358_Bus
  Bus Selector5 : BusSelector  OutputSignals=IO_CANInputs_Bus.IO_CAN1_Bus.IO_CAN1_PM100DX_Bus.IO_CAN1_160_Bus,IO_CANInputs_Bus.IO_CAN1_Bus.IO_CAN1_PM100DX_Bus.IO_CAN1_162_Bus,IO_CANInputs_Bus.IO_CAN1_Bus.IO_CAN1_PM100DX_Bus.IO_CAN1_165_Bus,IO_CANInputs_Bus.IO_CAN1_Bus.IO_CAN1_PM100DX_Bus.IO_CAN1_166_Bus,IO_CANInputs_Bus.IO_CAN1_Bus.IO_CAN1_PM100DX_Bus.IO_CAN1_167_Bus,IO_CANInputs_Bus.IO_CAN1_Bus.IO_CAN1_PM100DX_Bus.IO_CAN1_172_Bus
  Bus Selector6 : BusSelector  OutputSignals=IO_CANInputs_Bus.IO_CAN1_Bus.IO_CAN1_LWS_Bus.IO_CAN1_688_Bus
  Bus Selector7 : BusSelector  OutputSignals=IO_CANInputs_Bus.IO_CAN1_Bus.IO_CAN1_DCDC_Bus
  Bus Selector8 : BusSelector  OutputSignals=IO_CANInputs_Bus.IO_CAN2_Bus.IO_CAN2_MM5_Bus.IO_CAN2_372_Bus,IO_CANInputs_Bus.IO_CAN2_Bus.IO_CAN2_MM5_Bus.IO_CAN2_376_Bus,IO_CANInputs_Bus.IO_CAN2_Bus.IO_CAN2_MM5_Bus.IO_CAN2_380_Bus,IO_CANInputs_Bus.IO_CAN2_Bus.IO_CAN2_MM5_Bus.IO_CAN2_450_Bus,IO_CANInputs_Bus.IO_CAN2_Bus.IO_CAN2_MM5_Bus.IO_CAN2_451Bus
  IN_BrakePressure : BrakePressure/IN_BrakePressure  pos='F'
  IN_BrakePressure1 : BrakePressure/IN_BrakePressure  pos='R'
  IN_DCDC : DCDC/IN_DCDC  SystemSampleTime=-1  VariantActivationTime=update diagram  EmptyChoice=off  PassThrough=off  PassThroughVariantControl=(default)  EmptyChoiceVariantControl=(default)  AllowFlexibleInterface=on  Latency=0  AutoFrameSizeCalculation=off
  IN_TCDial : TCDial/IN_TCDial  pos=''
  IN_ThrottlePosition : ThrottlePosition/IN_ThrottlePosition  pos='1'
  IN_ThrottlePosition1 : ThrottlePosition/IN_ThrottlePosition  pos='2'
  LWS : LWS/LWS  SystemSampleTime=-1  VariantActivationTime=update diagram  EmptyChoice=off  PassThrough=off  PassThroughVariantControl=(default)  EmptyChoiceVariantControl=(default)  AllowFlexibleInterface=on  Latency=0  AutoFrameSizeCalculation=off
  MM5 : MM5/MM5  SystemSampleTime=-1  VariantActivationTime=update diagram  EmptyChoice=off  PassThrough=off  PassThroughVariantControl=(default)  EmptyChoiceVariantControl=(default)  AllowFlexibleInterface=on  Latency=0  AutoFrameSizeCalculation=off
  PM100DX : PM100DX/IN_PM100DX  SystemSampleTime=-1  VariantActivationTime=update diagram  EmptyChoice=off  PassThrough=off  PassThroughVariantControl=(default)  EmptyChoiceVariantControl=(default)  AllowFlexibleInterface=on  Latency=0  AutoFrameSizeCalculation=off
  IN_Inputs_Bus : Outport
  wires:
  IO_Inputs_Bus/1 -> [IO_Inputs_Bus]
  [IO_Inputs_Bus] -> Bus Selector/1
  Bus Selector/1 -> IN_TCDial/1  "<IO_TCKnob_V>"
  IN_TCDial/1 -> [IN_TCDial_na]  "IN_TCDial_na"
  [IO_Inputs_Bus] -> Bus Selector1/1
  IN_ThrottlePosition/1 -> Bus Creator/1  "IN_ThrottlePosition1_pct"
  IN_ThrottlePosition1/1 -> Bus Creator/2  "IN_ThrottlePosition2_pct"
  Bus Creator/1 -> [IN_ThrottlePosition_Bus]  "IN_ThrottlePosition_Bus"
  Bus Selector1/1 -> IN_ThrottlePosition/1  "<IO_ThrottlePosition1_V>"
  Bus Selector1/2 -> IN_ThrottlePosition1/1  "<IO_ThrottlePosition2_V>"
  Bus Creator1/1 -> [IN_BrakePressure_Bus]  "IN_BrakePressure_Bus"
  [IO_Inputs_Bus] -> Bus Selector2/1
  Bus Selector2/1 -> IN_BrakePressure/1  "<IO_BrakePressureF_V>"
  Bus Selector2/2 -> IN_BrakePressure1/1  "<IO_BrakePressureR_V>"
  IN_BrakePressure1/1 -> Bus Creator1/2  "IN_BrakePressureR_psi"
  IN_BrakePressure/1 -> Bus Creator1/1  "IN_BrakePressureF_psi"
  Bus Creator2/1 -> IN_Inputs_Bus/1
  [IO_Inputs_Bus] -> Bus Selector3/1
  Bus Selector3/1 -> ATCCF/1  "<IO_CAN1_301_Bus>"
  Bus Selector3/2 -> ATCCF/2  "<IO_CAN1_302_Bus>"
  Bus Selector3/3 -> ATCCF/3  "<IO_CAN1_303_Bus>"
  Bus Selector3/4 -> ATCCF/4  "<IO_CAN1_305_Bus>"
  [IO_Inputs_Bus] -> Bus Selector4/1
  Bus Selector4/1 -> ATCCR/1  "<IO_CAN1_351_Bus>"
  Bus Selector4/2 -> ATCCR/2  "<IO_CAN1_352_Bus>"
  Bus Selector4/3 -> ATCCR/3  "<IO_CAN1_353_Bus>"
  Bus Selector4/4 -> ATCCR/4  "<IO_CAN1_354_Bus>"
  Bus Selector4/5 -> ATCCR/5  "<IO_CAN1_355_Bus>"
  Bus Selector4/6 -> ATCCR/6  "<IO_CAN1_356_Bus>"
  Bus Selector4/7 -> ATCCR/7  "<IO_CAN1_357_Bus>"
  Bus Selector4/8 -> ATCCR/8  "<IO_CAN1_358_Bus>"
  [IO_Inputs_Bus] -> Bus Selector5/1
  Bus Selector5/1 -> PM100DX/1  "<IO_CAN1_160_Bus>"
  Bus Selector5/2 -> PM100DX/2  "<IO_CAN1_162_Bus>"
  Bus Selector5/3 -> PM100DX/3  "<IO_CAN1_165_Bus>"
  Bus Selector5/4 -> PM100DX/4  "<IO_CAN1_166_Bus>"
  Bus Selector5/5 -> PM100DX/5  "<IO_CAN1_167_Bus>"
  Bus Selector5/6 -> PM100DX/6  "<IO_CAN1_172_Bus>"
  ATCCF/1 -> [IN_CAN1_ATCCF_Bus]  "IN_CAN1_ATCCF_Bus"
  ATCCR/1 -> [IN_CAN1_ATCCR_Bus]  "IN_CAN1_ATCCR_Bus"
  [IO_Inputs_Bus] -> Bus Selector6/1
  Bus Selector6/1 -> LWS/1  "<IO_CAN1_688_Bus>"
  PM100DX/1 -> Bus Creator3/1  "IN_ModuleATemp_degC"
  PM100DX/2 -> Bus Creator3/2  "IN_ModuleBTemp_degC"
  PM100DX/3 -> Bus Creator3/3  "IN_ModuleCTemp_degC"
  PM100DX/4 -> Bus Creator3/4  "IN_MotorTemp_degC"
  PM100DX/5 -> Bus Creator3/5  "IN_MotorSpeed_rpm"
  PM100DX/6 -> Bus Creator3/6  "IN_DCBusCurrent_A"
  PM100DX/7 -> Bus Creator3/7  "IN_DCBusVoltage_V"
  PM100DX/8 -> Bus Creator3/8  "IN_TorqueFeedback_Nm"
  Bus Creator3/1 -> [IN_CAN1_PM100DX_Bus]
  [IO_Inputs_Bus] -> Bus Selector7/1
  Bus Selector7/1 -> IN_DCDC/1  "<IO_CAN1_DCDC_Bus>"
  LWS/1 -> Bus Creator4/1  "IN_SteeringAngle_deg"
  LWS/2 -> Bus Creator4/2  "IN_SteeringSpeed_degps"
  Bus Creator4/1 -> [IN_CAN1_LWS_Bus]
  IN_DCDC/1 -> Bus Creator5/1  "IN_CANError_en"
  IN_DCDC/2 -> Bus Creator5/2  "IN_CurrentOutput_A"
  IN_DCDC/3 -> Bus Creator5/3  "IN_HardwareFault_en"
  IN_DCDC/4 -> Bus Creator5/4  "IN_HVILError_en"
  IN_DCDC/5 -> Bus Creator5/5  "IN_InputOverVoltage_en"
  IN_DCDC/6 -> Bus Creator5/6  "IN_InputUnderVoltage_en"
  IN_DCDC/7 -> Bus Creator5/7  "IN_OutputOverCurrent_en"
  IN_DCDC/8 -> Bus Creator5/8  "IN_OutputOverVoltage_en"
  IN_DCDC/9 -> Bus Creator5/9  "IN_OutputUnderVoltage_en"
  IN_DCDC/10 -> Bus Creator5/10  "IN_OverTempError_en"
  IN_DCDC/11 -> Bus Creator5/11  "IN_DCDCReady_en"
  IN_DCDC/12 -> Bus Creator5/12  "IN_ShutOffError_en"
  IN_DCDC/13 -> Bus Creator5/13  "IN_DCDCStatus_en"
  IN_DCDC/14 -> Bus Creator5/14  "IN_TempWarning_en"
  IN_DCDC/15 -> Bus Creator5/15  "IN_Temperature_degC"
  IN_DCDC/16 -> Bus Creator5/16  "IN_VoltageOutput_V"
  Bus Creator5/1 -> [IN_CAN1_DCDC_Bus]  "IN_CAN1_DCDC_Bus"
  MM5/1 -> Bus Creator6/1  "IN_MM51Ay_g"
  MM5/2 -> Bus Creator6/2  "IN_MM51YawRate_na"
  MM5/3 -> Bus Creator6/3  "IN_MM51Ax_g"
  MM5/4 -> Bus Creator6/4  "IN_MM51RollRate_na"
  MM5/5 -> Bus Creator6/5  "IN_MM51Az_g"
  MM5/6 -> Bus Creator6/6  "IN_MM52Ay_g"
  MM5/7 -> Bus Creator6/7  "IN_MM52YawRate_na"
  MM5/8 -> Bus Creator6/8  "IN_MM52Ax_g"
  MM5/9 -> Bus Creator6/9  "IN_MM52Az_g"
  MM5/10 -> Bus Creator6/10  "IN_MM52RollRate_na"
  [IN_TCDial_na] -> Bus Creator2/1  "IN_TCDial_na"
  [IN_ThrottlePosition_Bus] -> Bus Creator2/2  "IN_ThrottlePosition_Bus"
  [IN_BrakePressure_Bus] -> Bus Creator2/3  "IN_BrakePressure_Bus"
  [IN_CAN1_ATCCF_Bus] -> Bus Creator2/4  "IN_CAN1_ATCCF_Bus"
  [IN_CAN1_ATCCR_Bus] -> Bus Creator2/5  "IN_CAN1_ATCCR_Bus"
  [IN_CAN1_PM100DX_Bus] -> Bus Creator2/6  "IN_CAN1_PM100DX_Bus"
  [IN_CAN1_LWS_Bus] -> Bus Creator2/7  "IN_CAN1_LWS_Bus"
  [IN_CAN1_DCDC_Bus] -> Bus Creator2/8  "IN_CAN1_DCDC_Bus"
  [IN_CAN2_MM5_Bus] -> Bus Creator2/9  "IN_CAN2_MM5_Bus"
  Bus Selector8/1 -> MM5/1  "<IO_CAN2_372_Bus>"
  Bus Selector8/2 -> MM5/2  "<IO_CAN2_376_Bus>"
  Bus Selector8/3 -> MM5/3  "<IO_CAN2_380_Bus>"
  Bus Selector8/4 -> MM5/4  "<IO_CAN2_450_Bus>"
  Bus Selector8/5 -> MM5/5  "<IO_CAN2_451Bus>"
  [IO_Inputs_Bus] -> Bus Selector8/1
  Bus Creator6/1 -> [IN_CAN2_MM5_Bus]

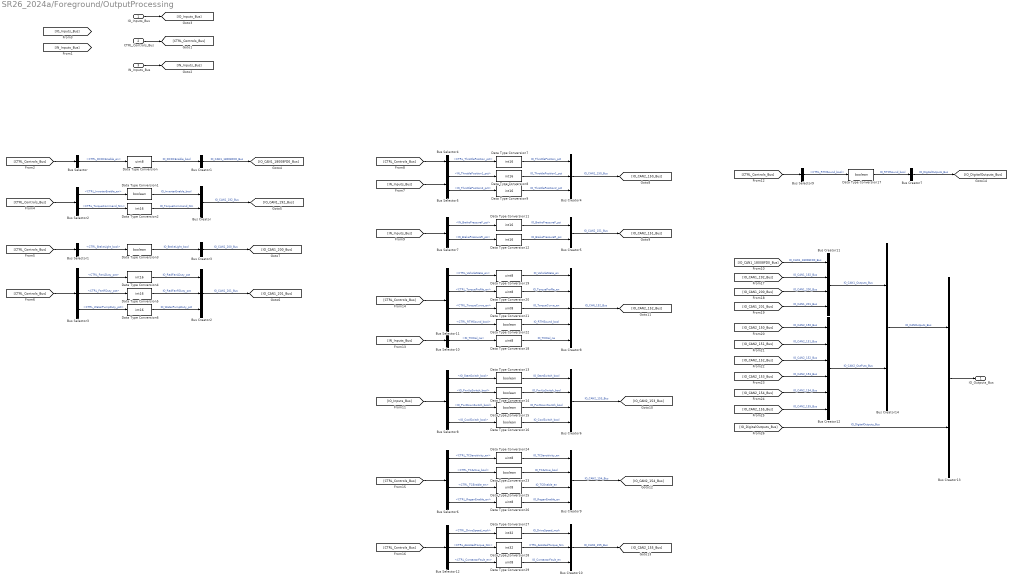
== system SR26_2024a/Foreground/OutputProcessing ==
  IO_Inputs_Bus : Inport
  CTRL_Controls_Bus : Inport  Port=2
  IN_Inputs_Bus : Inport  Port=3
  Bus Creator{,5,13..14} (4 alike) : BusCreator  Inputs=2
  Bus Creator1 : BusCreator  Inputs=1
  Bus Creator10 : BusCreator  Inputs=3
  Bus Creator11 : BusCreator  Inputs=4
  Bus Creator12 : BusCreator  Inputs=6
  Bus Creator2 : BusCreator  Inputs=3
  Bus Creator3 : BusCreator  Inputs=1
  Bus Creator4 : BusCreator  Inputs=3
  Bus Creator6 : BusCreator  Inputs=4
  Bus Creator7 : BusCreator  Inputs=1
  Bus Creator8 : BusCreator  Inputs=5
  Bus Creator9 : BusCreator  Inputs=4
  Bus Selector : BusSelector  OutputSignals=CTRL_DCDCEnable_en
  Bus Selector1 : BusSelector  OutputSignals=CTRL_BrakeLight_bool
  Bus Selector10 : BusSelector  OutputSignals=IN_TCDial_na
  Bus Selector11 : BusSelector  OutputSignals=CTRL_VehicleState_en,CTRL_TorqueProfile_en,CTRL_TorqueCurve_en,CTRL_RTMSound_bool
  Bus Selector12 : BusSelector  OutputSignals=CTRL_DriveSpeed_mph,CTRL_AssistedTorque_Nm,CTRL_ContactorFault_en
  Bus Selector2 : BusSelector  OutputSignals=CTRL_InverterEnable_en,CTRL_TorqueCommand_Nm
  Bus Selector3 : BusSelector  OutputSignals=CTRL_FanLDuty_pct,CTRL_FanRDuty_pct,CTRL_WaterPumpDuty_pct
  Bus Selector4 : BusSelector  OutputSignals=CTRL_ThrottlePosition_pct
  Bus Selector5 : BusSelector  OutputSignals=IN_ThrottlePosition_Bus.IN_ThrottlePosition1_pct,IN_ThrottlePosition_Bus.IN_ThrottlePosition2_pct
  Bus Selector6 : BusSelector  OutputSignals=CTRL_TCSensitivity_en,CTRL_TCActive_bool,CTRL_TCEnable_en,CTRL_RegenEnable_en
  Bus Selector7 : BusSelector  OutputSignals=IN_BrakePressure_Bus.IN_BrakePressureF_psi,IN_BrakePressure_Bus.IN_BrakePressureR_psi
  Bus Selector8 : BusSelector  OutputSignals=IO_DigitalInputs_Bus.IO_StartSwitch_bool,IO_DigitalInputs_Bus.IO_PwrUpSwitch_bool,IO_DigitalInputs_Bus.IO_PwrDownSwitch_bool,IO_DigitalInputs_Bus.IO_CoolSwitch_bool
  Bus Selector9 : BusSelector  OutputSignals=CTRL_RTMSound_bool
  Data Type Conversion{,18..21,24..26,29} (9 alike) : DataTypeConversion  OutDataTypeStr=uint8  SaturateOnIntegerOverflow=off  RndMeth=Floor
  Data Type Conversion{1,3,13..17,22..23} (9 alike) : DataTypeConversion  OutDataTypeStr=boolean  SaturateOnIntegerOverflow=off  RndMeth=Floor
  Data Type Conversion{2,4..9,11..12} (9 alike) : DataTypeConversion  OutDataTypeStr=int16  SaturateOnIntegerOverflow=off  RndMeth=Floor
  Data Type Conversion27 : DataTypeConversion  OutDataTypeStr=int32  SaturateOnIntegerOverflow=off  RndMeth=Floor
  Data Type Conversion28 : DataTypeConversion  OutDataTypeStr=int32  SaturateOnIntegerOverflow=off  RndMeth=Floor
  IO_Outputs_Bus : Outport
  wires:
  IO_Inputs_Bus/1 -> [IO_Inputs_Bus]
  CTRL_Controls_Bus/1 -> [CTRL_Controls_Bus]
  IN_Inputs_Bus/1 -> [IN_Inputs_Bus]
  [CTRL_Controls_Bus] -> Bus Selector/1
  Bus Selector/1 -> Data Type Conversion/1  "<CTRL_DCDCEnable_en>"
  Bus Creator1/1 -> [IO_CAN1_18008FD0_Bus]  "IO_CAN1_18008FD0_Bus"
  [CTRL_Controls_Bus] -> Bus Selector2/1
  Bus Selector2/1 -> Data Type Conversion1/1  "<CTRL_InverterEnable_en>"
  Bus Selector2/2 -> Data Type Conversion2/1  "<CTRL_TorqueCommand_Nm>"
  Data Type Conversion2/1 -> Bus Creator/2  "IO_TorqueCommand_Nm"
  Data Type Conversion1/1 -> Bus Creator/1  "IO_InverterEnable_bool"
  Data Type Conversion/1 -> Bus Creator1/1  "IO_DCDCEnable_bool"
  Bus Creator/1 -> [IO_CAN1_192_Bus]  "IO_CAN1_192_Bus"
  [CTRL_Controls_Bus] -> Bus Selector1/1
  Bus Selector1/1 -> Data Type Conversion3/1  "<CTRL_BrakeLight_bool>"
  [CTRL_Controls_Bus] -> Bus Selector3/1
  Bus Selector3/1 -> Data Type Conversion4/1  "<CTRL_FanLDuty_pct>"
  Bus Selector3/2 -> Data Type Conversion5/1  "<CTRL_FanRDuty_pct>"
  Bus Selector3/3 -> Data Type Conversion6/1  "<CTRL_WaterPumpDuty_pct>"
  Data Type Conversion4/1 -> Bus Creator2/1  "IO_RadFanLDuty_pct"
  Data Type Conversion5/1 -> Bus Creator2/2  "IO_RadFanRDuty_pct"
  Data Type Conversion6/1 -> Bus Creator2/3  "IO_WaterPumpDuty_pct"
  Bus Creator2/1 -> [IO_CAN1_201_Bus]  "IO_CAN1_201_Bus"
  Data Type Conversion3/1 -> Bus Creator3/1  "IO_BrakeLight_bool"
  Bus Creator3/1 -> [IO_CAN1_200_Bus]  "IO_CAN1_200_Bus"
  [CTRL_Controls_Bus] -> Bus Selector4/1
  Bus Selector4/1 -> Data Type Conversion7/1  "<CTRL_ThrottlePosition_pct>"
  Data Type Conversion7/1 -> Bus Creator4/1  "IO_ThrottlePosition_pct"
  Bus Creator4/1 -> [IO_CAN2_150_Bus]  "IO_CAN1_150_Bus"
  [IN_Inputs_Bus] -> Bus Selector5/1
  Bus Selector5/1 -> Data Type Conversion8/1  "<IN_ThrottlePosition1_pct>"
  Bus Selector5/2 -> Data Type Conversion9/1  "<IN_ThrottlePosition2_pct>"
  Data Type Conversion8/1 -> Bus Creator4/2  "IO_ThrottlePosition1_pct"
  Data Type Conversion9/1 -> Bus Creator4/3  "IO_ThrottlePosition2_pct"
  Data Type Conversion12/1 -> Bus Creator5/2  "IO_BrakePressureR_psi"
  Data Type Conversion11/1 -> Bus Creator5/1  "IO_BrakePressureF_psi"
  [IN_Inputs_Bus] -> Bus Selector7/1
  Bus Creator5/1 -> [IO_CAN2_151_Bus]  "IO_CAN2_151_Bus"
  Bus Selector7/1 -> Data Type Conversion11/1  "<IN_BrakePressureF_psi>"
  Bus Selector7/2 -> Data Type Conversion12/1  "<IN_BrakePressureR_psi>"
  [IO_Inputs_Bus] -> Bus Selector8/1
  Bus Selector8/4 -> Data Type Conversion16/1  "<IO_CoolSwitch_bool>"
  Bus Selector8/3 -> Data Type Conversion15/1  "<IO_PwrDownSwitch_bool>"
  Bus Selector8/2 -> Data Type Conversion14/1  "<IO_PwrUpSwitch_bool>"
  Bus Selector8/1 -> Data Type Conversion13/1  "<IO_StartSwitch_bool>"
  Data Type Conversion13/1 -> Bus Creator6/1  "IO_StartSwitch_bool"
  Data Type Conversion14/1 -> Bus Creator6/2  "IO_PwrUpSwitch_bool"
  Data Type Conversion15/1 -> Bus Creator6/3  "IO_PwrDownSwitch_bool"
  Data Type Conversion16/1 -> Bus Creator6/4  "IO_CoolSwitch_bool"
  Bus Creator6/1 -> [IO_CAN2_153_Bus]  "IO_CAN2_153_Bus"
  [CTRL_Controls_Bus] -> Bus Selector9/1
  Bus Selector9/1 -> Data Type Conversion17/1  "<CTRL_RTMSound_bool>"
  Data Type Conversion17/1 -> Bus Creator7/1  "IO_RTMSound_bool"
  Bus Creator7/1 -> [IO_DigitalOutputs_Bus]  "IO_DigitalOutputs_Bus"
  Bus Creator8/1 -> [IO_CAN2_152_Bus]  "IO_CAN_152_Bus"
  Bus Selector10/1 -> Data Type Conversion18/1  "<IN_TCDial_na>"
  [IN_Inputs_Bus] -> Bus Selector10/1
  [CTRL_Controls_Bus] -> Bus Selector11/1
  Bus Selector11/1 -> Data Type Conversion19/1  "<CTRL_VehicleState_en>"
  Bus Selector11/2 -> Data Type Conversion20/1  "<CTRL_TorqueProfile_en>"
  Bus Selector11/3 -> Data Type Conversion21/1  "<CTRL_TorqueCurve_en>"
  Bus Selector11/4 -> Data Type Conversion22/1  "<CTRL_RTMSound_bool>"
  Data Type Conversion19/1 -> Bus Creator8/1  "IO_VehicleState_en"
  Data Type Conversion20/1 -> Bus Creator8/2  "IO_TorqueProfile_en"
  Data Type Conversion21/1 -> Bus Creator8/3  "IO_TorqueCurve_en"
  Data Type Conversion22/1 -> Bus Creator8/4  "IO_RTMSound_bool"
  Data Type Conversion18/1 -> Bus Creator8/5  "IO_TCDial_na"
  [CTRL_Controls_Bus] -> Bus Selector6/1
  Bus Selector6/1 -> Data Type Conversion24/1  "<CTRL_TCSensitivity_en>"
  Bus Selector6/2 -> Data Type Conversion23/1  "<CTRL_TCActive_bool>"
  Bus Selector6/3 -> Data Type Conversion25/1  "<CTRL_TCEnable_en>"
  Bus Selector6/4 -> Data Type Conversion26/1  "<CTRL_RegenEnable_en>"
  Data Type Conversion23/1 -> Bus Creator9/2  "IO_TCActive_bool"
  Data Type Conversion24/1 -> Bus Creator9/1  "IO_TCSensitivity_en"
  Data Type Conversion25/1 -> Bus Creator9/3  "IO_TCEnable_en"
  Data Type Conversion26/1 -> Bus Creator9/4  "IO_RegenEnable_en"
  Bus Creator9/1 -> [IO_CAN2_154_Bus]  "IO_CAN2_154_Bus"
  [CTRL_Controls_Bus] -> Bus Selector12/1
  Bus Selector12/1 -> Data Type Conversion27/1  "<CTRL_DriveSpeed_mph>"
  Bus Selector12/2 -> Data Type Conversion28/1  "<CTRL_AssistedTorque_Nm>"
  Bus Selector12/3 -> Data Type Conversion29/1  "<CTRL_ContactorFault_en>"
  Data Type Conversion29/1 -> Bus Creator10/3  "IO_ContactorFault_en"
  Data Type Conversion28/1 -> Bus Creator10/2  "CTRL_AssistedTorque_Nm"
  Data Type Conversion27/1 -> Bus Creator10/1  "IO_DriveSpeed_mph"
  Bus Creator10/1 -> [IO_CAN2_155_Bus]  "IO_CAN2_155_Bus"
  [IO_CAN1_18008FD0_Bus] -> Bus Creator11/1  "IO_CAN1_18008FD0_Bus"
  [IO_CAN1_192_Bus] -> Bus Creator11/2  "IO_CAN1_192_Bus"
  [IO_CAN1_200_Bus] -> Bus Creator11/3  "IO_CAN1_200_Bus"
  [IO_CAN1_201_Bus] -> Bus Creator11/4  "IO_CAN1_201_Bus"
  [IO_CAN2_150_Bus] -> Bus Creator12/1  "IO_CAN2_150_Bus"
  [IO_CAN2_151_Bus] -> Bus Creator12/2  "IO_CAN2_151_Bus"
  [IO_CAN2_152_Bus] -> Bus Creator12/3  "IO_CAN2_152_Bus"
  [IO_CAN2_153_Bus] -> Bus Creator12/4  "IO_CAN2_153_Bus"
  [IO_CAN2_154_Bus] -> Bus Creator12/5  "IO_CAN2_154_Bus"
  [IO_CAN2_155_Bus] -> Bus Creator12/6  "IO_CAN2_155_Bus"
  [IO_DigitalOutputs_Bus] -> Bus Creator13/2  "IO_DigitalOutputs_Bus"
  Bus Creator13/1 -> IO_Outputs_Bus/1
  Bus Creator11/1 -> Bus Creator14/1  "IO_CAN1_Outputs_Bus"
  Bus Creator12/1 -> Bus Creator14/2  "IO_CAN2_OutPuts_Bus"
  Bus Creator14/1 -> Bus Creator13/1  "IO_CANOutputs_Bus"
